simulink model "magDesat_test"  (R2018b)
settings: Solver=VariableStepAuto  StartTime=0.0  StopTime=2000  RelTol=1e-3
undefined symbols (not defined in the file or in its folder): DiscIntNeverNeededParam, fswParams, reaction_wheel_assembly_lib, simParams
libraries: reaction_wheel_PID_lib x4, rw_motor_lib x4, vrlib x2, Desaturation_Controller_lib x1, Detumbling_Controller_lib x1, aerolibutil x1, sharedutil x1
settings Model: Creator=colem  LastModifiedBy=colem

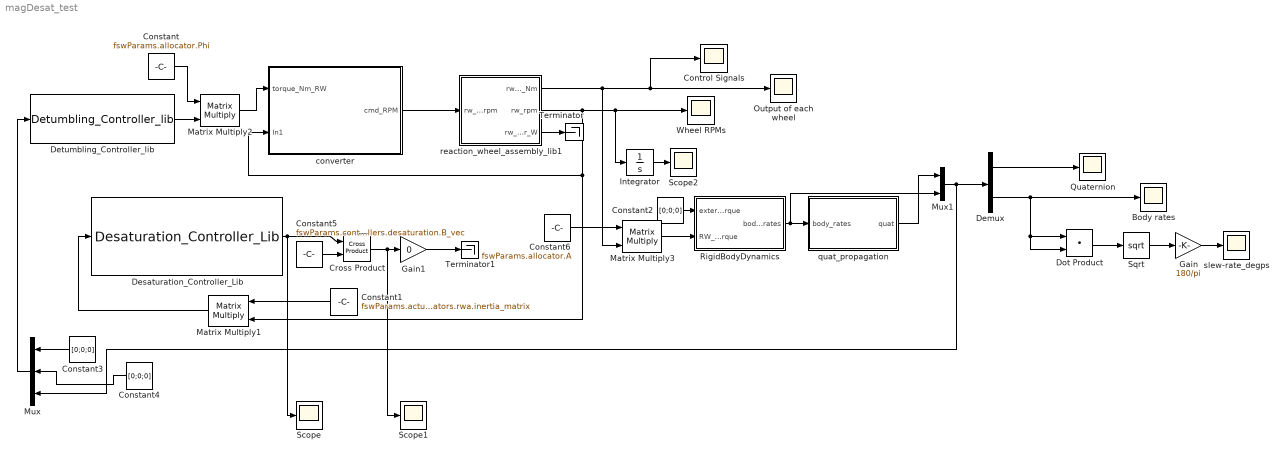
== system magDesat_test ==
  Body rates : Scope
  Constant : Constant  Value=fswParams.allocator.Phi
  Constant1 : Constant  Value=fswParams.actuators.rwa.inertia_matrix
  Constant2 : Constant  Value=[0;0;0]
  Constant3 : Constant  Value=[0;0;0]
  Constant4 : Constant  Value=[0;0;0]
  Constant5 : Constant  Value=fswParams.controllers.desaturation.B_vec
  Constant6 : Constant  Value=fswParams.allocator.A
  Control Signals : Scope
  Cross Product : vrlib/Utilities/Cross Product
      settings: SourceProductBaseCode=VR
  Demux : Demux  Outputs=[4 3]
  Desaturation_Controller_Lib : Desaturation_Controller_lib/Desaturation_Controller_Lib  SystemSampleTime=-1
  Detumbling_Controller_lib : Detumbling_Controller_lib/Detumbling_Controller_lib  SystemSampleTime=-1
  Dot Product : DotProduct  InputSameDT=on  OutDataTypeStr=Inherit: Inherit via internal rule
  Gain : Gain  Gain=180/pi
  Gain1 : Gain  Gain=0
  Integrator : Integrator
  Matrix Multiply1 : Product  Multiplication=Matrix(*)
  Matrix Multiply2 : Product  Multiplication=Matrix(*)
  Matrix Multiply3 : Product  Multiplication=Matrix(*)
  Mux : Mux  Inputs=[3 3 7]
  Mux1 : Mux  Inputs=[4 3]
  Output of each wheel : Scope
  Quaternion : Scope
  RigidBodyDynamics : Subsystem
  Scope : Scope
  Scope1 : Scope
  Scope2 : Scope
  Sqrt : Sqrt  SaturateOnIntegerOverflow=on
  Terminator : Terminator
  Terminator1 : Terminator
  Wheel RPMs : Scope
  converter : Subsystem
  quat_propagation : Subsystem
  reaction_wheel_assembly_lib1 : Subsystem  AncestorBlock=reaction_wheel_assembly_lib/reaction_wheel_assembly_lib
  slew-rate_degps : Scope
  wires:
  Demux/1 -> Quaternion/1
  reaction_wheel_assembly_lib1/1(rw_torque_Nm) -> Control Signals/1, Output of each wheel/1, Matrix Multiply3/2
  Mux1/1 -> Demux/1, Mux/3
  Constant3/1 -> Mux/1
  Constant4/1 -> Mux/2
  Mux/1 -> Detumbling_Controller_lib/1
  Demux/2 -> Body rates/1, Dot Product/2, Dot Product/1
  Sqrt/1 -> Gain/1
  Gain/1 -> slew-rate_degps/1
  Dot Product/1 -> Sqrt/1
  Desaturation_Controller_Lib/1 -> Scope/1, Cross Product/1
  Constant1/1 -> Matrix Multiply1/1
  Matrix Multiply1/1 -> Desaturation_Controller_Lib/1
  reaction_wheel_assembly_lib1/3(rw_power_W) -> Terminator/1
  Constant5/1 -> Cross Product/2
  Detumbling_Controller_lib/1 -> Matrix Multiply2/2
  Matrix Multiply2/1 -> converter/1(torque_Nm_RW)
  Constant/1 -> Matrix Multiply2/1
  Cross Product/1 -> Scope1/1, Gain1/1
  RigidBodyDynamics/1(body_rates) -> quat_propagation/1(body_rates), Mux1/2
  quat_propagation/1(quat) -> Mux1/1
  Constant6/1 -> Matrix Multiply3/1
  Matrix Multiply3/1 -> RigidBodyDynamics/2(RW_torque)
  converter/1(cmd_RPM) -> reaction_wheel_assembly_lib1/1(rw_cmd_rpm)
  Gain1/1 -> Terminator1/1
  Constant2/1 -> RigidBodyDynamics/1(external_torque)
  reaction_wheel_assembly_lib1/2(rw_rpm) -> converter/2(In1), Matrix Multiply1/2, Integrator/1, Wheel RPMs/1
  Integrator/1 -> Scope2/1

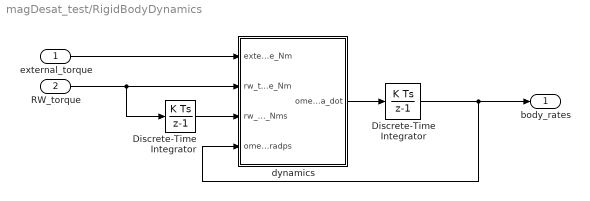
== system magDesat_test/RigidBodyDynamics ==
  external_torque : Inport
  RW_torque : Inport  Port=2
  Discrete-Time Integrator : DiscreteIntegrator  InitialCondition=[0;0;0]  SampleTime=-1  ICPrevOutput=DiscIntNeverNeededParam  ICPrevScaledInput=DiscIntNeverNeededParam
  "Discrete-Time Integrator " : DiscreteIntegrator  InitialCondition=[1;1;1]*.5  SampleTime=-1  ICPrevOutput=DiscIntNeverNeededParam  ICPrevScaledInput=DiscIntNeverNeededParam
  dynamics : Subsystem
  body_rates : Outport
  wires:
  RW_torque/1 -> dynamics/2(rw_torque_Nm), Discrete-Time Integrator/1
  Discrete-Time Integrator/1 -> dynamics/3(rw_momentum_Nms)
  "Discrete-Time Integrator "/1 -> body_rates/1, dynamics/4(omega_radps)
  external_torque/1 -> dynamics/1(external_torque_Nm)
  dynamics/1(omega_dot) -> "Discrete-Time Integrator "/1

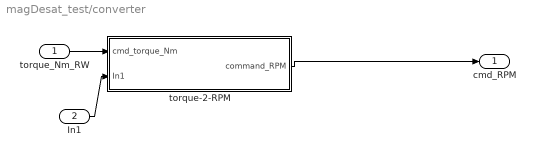
== system magDesat_test/converter ==
  torque_Nm_RW : Inport
  In1 : Inport  Port=2
  torque-2-RPM : Subsystem
  cmd_RPM : Outport
  wires:
  torque_Nm_RW/1 -> torque-2-RPM/1(cmd_torque_Nm)
  torque-2-RPM/1(command_RPM) -> cmd_RPM/1
  In1/1 -> torque-2-RPM/2(In1)

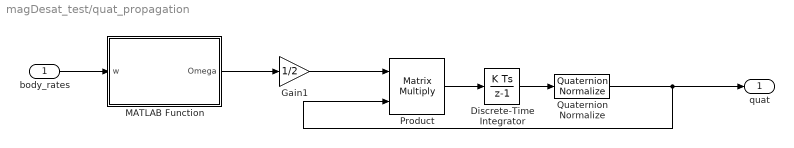
== system magDesat_test/quat_propagation ==
  body_rates : Inport
  Discrete-Time Integrator : DiscreteIntegrator  InitialCondition=simParams.initialConditions.q0  SampleTime=-1  ICPrevOutput=DiscIntNeverNeededParam  ICPrevScaledInput=DiscIntNeverNeededParam
  Gain1 : Gain  Gain=1/2
  MATLAB Function : MATLAB Function  TreatAsAtomicUnit=on
  Product : Product  Multiplication=Matrix(*)  RndMeth=Zero
  Quaternion Normalize : sharedutil/Quaternion Normalize  aMode=aMode
      settings: SourceProductName=Aerospace Blockset  SourceProductBaseCode=AE
  quat : Outport
  wires:
  Product/1 -> Discrete-Time Integrator/1
  Discrete-Time Integrator/1 -> Quaternion Normalize/1
  Gain1/1 -> Product/1
  Quaternion Normalize/1 -> quat/1, Product/2
  body_rates/1 -> MATLAB Function/1(w)
  MATLAB Function/1(Omega) -> Gain1/1

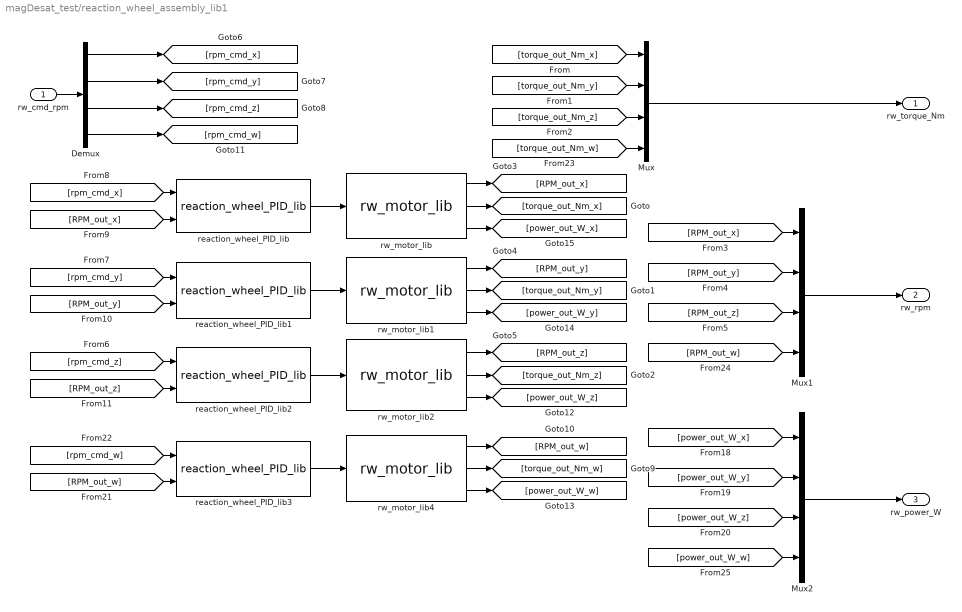
== system magDesat_test/reaction_wheel_assembly_lib1 ==
  rw_cmd_rpm : Inport
  Demux : Demux
  Mux : Mux
  Mux1 : Mux
  Mux2 : Mux
  reaction_wheel_PID_lib{,1..3} (4 alike) : reaction_wheel_PID_lib/reaction_wheel_PID_lib  SystemSampleTime=-1
  rw_motor_lib{,1..2,4} (4 alike) : rw_motor_lib/rw_motor_lib  SystemSampleTime=-1
  rw_torque_Nm : Outport
  rw_rpm : Outport  Port=2
  rw_power_W : Outport  Port=3
  wires:
  [power_out_W_w] -> Mux2/4
  [power_out_W_z] -> Mux2/3
  [power_out_W_y] -> Mux2/2
  [power_out_W_x] -> Mux2/1
  [RPM_out_w] -> Mux1/4
  [torque_out_Nm_w] -> Mux/4
  rw_motor_lib/3 -> [power_out_W_x]
  rw_motor_lib1/3 -> [power_out_W_y]
  Demux/4 -> [rpm_cmd_w]
  rw_motor_lib4/3 -> [power_out_W_w]
  [RPM_out_w] -> reaction_wheel_PID_lib3/2
  reaction_wheel_PID_lib3/1 -> rw_motor_lib4/1
  rw_motor_lib4/1 -> [RPM_out_w]
  [rpm_cmd_w] -> reaction_wheel_PID_lib3/1
  rw_motor_lib4/2 -> [torque_out_Nm_w]
  Mux2/1 -> rw_power_W/1
  rw_motor_lib2/3 -> [power_out_W_z]
  reaction_wheel_PID_lib/1 -> rw_motor_lib/1
  Demux/1 -> [rpm_cmd_x]
  reaction_wheel_PID_lib1/1 -> rw_motor_lib1/1
  reaction_wheel_PID_lib2/1 -> rw_motor_lib2/1
  rw_cmd_rpm/1 -> Demux/1
  [torque_out_Nm_x] -> Mux/1
  [torque_out_Nm_y] -> Mux/2
  [torque_out_Nm_z] -> Mux/3
  rw_motor_lib1/2 -> [torque_out_Nm_y]
  rw_motor_lib2/2 -> [torque_out_Nm_z]
  [RPM_out_x] -> Mux1/1
  [RPM_out_y] -> Mux1/2
  [RPM_out_z] -> Mux1/3
  rw_motor_lib/2 -> [torque_out_Nm_x]
  rw_motor_lib/1 -> [RPM_out_x]
  rw_motor_lib2/1 -> [RPM_out_z]
  rw_motor_lib1/1 -> [RPM_out_y]
  [RPM_out_x] -> reaction_wheel_PID_lib/2
  [RPM_out_y] -> reaction_wheel_PID_lib1/2
  [RPM_out_z] -> reaction_wheel_PID_lib2/2
  Mux1/1 -> rw_rpm/1
  Demux/3 -> [rpm_cmd_z]
  Demux/2 -> [rpm_cmd_y]
  [rpm_cmd_z] -> reaction_wheel_PID_lib2/1
  [rpm_cmd_y] -> reaction_wheel_PID_lib1/1
  [rpm_cmd_x] -> reaction_wheel_PID_lib/1
  Mux/1 -> rw_torque_Nm/1

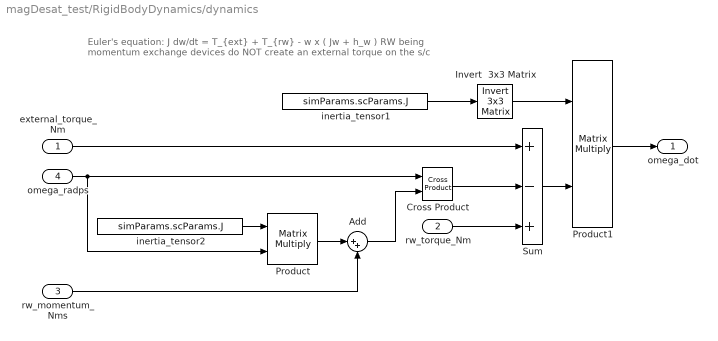
== system magDesat_test/RigidBodyDynamics/dynamics ==
  note: Euler's equation: J dw/dt = T_{ext} + T_{rw} - w x ( Jw + h_w )
      |
      | RW being momentum exchange devices do NOT create
      | an external torque on the s/c
  external_torque_Nm : Inport
  rw_torque_Nm : Inport  Port=2
  rw_momentum_Nms : Inport  Port=3
  omega_radps : Inport  Port=4
  Add : Sum  Inputs=|++
  Cross Product : vrlib/Utilities/Cross Product
      settings: SourceProductBaseCode=VR
  Invert  3x3 Matrix : aerolibutil/Invert  3x3 Matrix
  Product : Product  Multiplication=Matrix(*)  RndMeth=Zero
  Product1 : Product  Multiplication=Matrix(*)  RndMeth=Zero
  Sum : Sum  Inputs=+-+
  inertia_tensor1 : Constant  Value=simParams.scParams.J  SampleTime=simParams.sample_time_s
  inertia_tensor2 : Constant  Value=simParams.scParams.J  SampleTime=simParams.sample_time_s
  omega_dot : Outport
  wires:
  rw_torque_Nm/1 -> Sum/3
  Add/1 -> Cross Product/2
  Product/1 -> Add/1
  Cross Product/1 -> Sum/2
  inertia_tensor1/1 -> Invert  3x3 Matrix/1
  Invert  3x3 Matrix/1 -> Product1/1
  Product1/1 -> omega_dot/1
  Sum/1 -> Product1/2
  inertia_tensor2/1 -> Product/1
  omega_radps/1 -> Cross Product/1, Product/2
  external_torque_Nm/1 -> Sum/1
  rw_momentum_Nms/1 -> Add/2

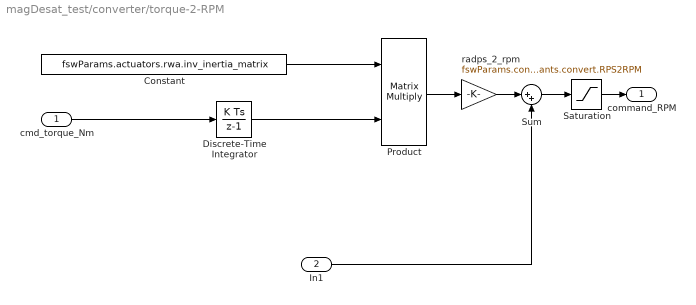
== system magDesat_test/converter/torque-2-RPM ==
  cmd_torque_Nm : Inport
  In1 : Inport  Port=2
  Constant : Constant  Value=fswParams.actuators.rwa.inv_inertia_matrix  SampleTime=fswParams.sample_time_s
  Discrete-Time Integrator : DiscreteIntegrator  SampleTime=-1  ICPrevOutput=DiscIntNeverNeededParam  ICPrevScaledInput=DiscIntNeverNeededParam
  Product : Product  Multiplication=Matrix(*)
  Saturation : Saturate  UpperLimit=fswParams.actuators.rwa.max_RPM  LowerLimit=-fswParams.actuators.rwa.max_RPM
  Sum : Sum  Inputs=|++
  radps_2_rpm : Gain  Gain=fswParams.constants.convert.RPS2RPM
  command_RPM : Outport
  wires:
  Saturation/1 -> command_RPM/1
  Discrete-Time Integrator/1 -> Product/2
  cmd_torque_Nm/1 -> Discrete-Time Integrator/1
  Product/1 -> radps_2_rpm/1
  Constant/1 -> Product/1
  radps_2_rpm/1 -> Sum/1
  Sum/1 -> Saturation/1
  In1/1 -> Sum/2

== matlab function magDesat_test/quat_propagation/MATLAB Function ==
  data: w input; Omega output
function Omega = skew_sym(w)
%#codegen

    w_skew = ...
        [0 w(3) -w(2);
        -w(3) 0 w(1);
        w(2) -w(1) 0];

    Omega = ...
        [0 -w';
        w w_skew];
